simulink model "flattening_3_test"  (Simulink 9.0)
settings: Solver=FixedStepAuto  StartTime=0.0  StopTime=10.0  FixedStep=1.000000  RelTol=1e-3  EnableMultiTasking=on
settings Model: SuppressorTable=22 serialization::archive 11 0 6 0 0 0 0 0  Creator=arnaud  LastModifiedBy=hbourbou
settings DataIOCC: LimitDataPoints=on  SignalLoggingSaveFormat=ModelDataLogs
settings OptimizationCC: ExpressionDepthLimit=2147483647
settings DebuggingCC: SolverPrmCheckMsg=warning  FcnCallInpInsideContextMsg=warning  StateNameClashWarn=warning  StrictBusMsg=Warning
settings GRTTargetCC: CombineOutputUpdateFcns=off  GRTInterface=on

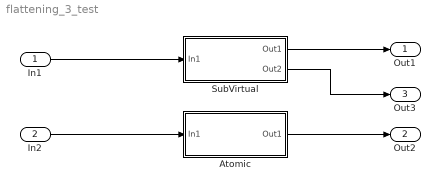
== system flattening_3_test ==
  In1 : Inport
  In2 : Inport  Port=2
  Atomic : Subsystem  TreatAsAtomicUnit=on
  SubVirtual : Subsystem
  Out1 : Outport
  Out2 : Outport  Port=2
  Out3 : Outport  Port=3
  wires:
  SubVirtual/1(Out1) -> Out1/1
  Atomic/1(Out1) -> Out2/1
  In1/1 -> SubVirtual/1(In1)
  In2/1 -> Atomic/1(In1)
  SubVirtual/2(Out2) -> Out3/1

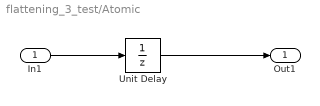
== system flattening_3_test/Atomic ==
  In1 : Inport
  Unit Delay : UnitDelay
  Out1 : Outport
  wires:
  In1/1 -> Unit Delay/1
  Unit Delay/1 -> Out1/1

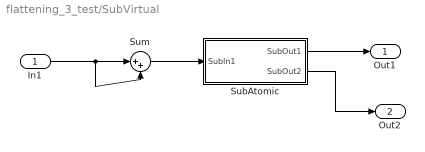
== system flattening_3_test/SubVirtual ==
  In1 : Inport
  SubAtomic : Subsystem  TreatAsAtomicUnit=on
  Sum : Sum  Inputs=|++
  Out1 : Outport
  Out2 : Outport  Port=2
  wires:
  SubAtomic/1(SubOut1) -> Out1/1
  Sum/1 -> SubAtomic/1(SubIn1)
  In1/1 -> Sum/1, Sum/2
  SubAtomic/2(SubOut2) -> Out2/1

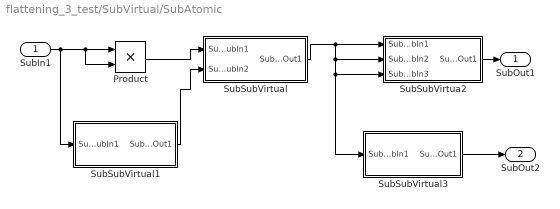
== system flattening_3_test/SubVirtual/SubAtomic ==
  SubIn1 : Inport
  Product : Product  RndMeth=Zero
  SubSubVirtua2 : Subsystem
  SubSubVirtual : Subsystem
  SubSubVirtual1 : Subsystem
  SubSubVirtual3 : Subsystem
  SubOut1 : Outport
  SubOut2 : Outport  Port=2
  wires:
  SubSubVirtual/1(SubSubOut1) -> SubSubVirtua2/1(SubSubIn1), SubSubVirtua2/2(SubSubIn2), SubSubVirtua2/3(SubSubIn3), SubSubVirtual3/1(SubSubIn1)
  Product/1 -> SubSubVirtual/1(SubSubIn1)
  SubIn1/1 -> Product/1, Product/2, SubSubVirtual1/1(SubSubIn1)
  SubSubVirtual1/1(SubSubOut1) -> SubSubVirtual/2(SubSubIn2)
  SubSubVirtua2/1(SubSubOut1) -> SubOut1/1
  SubSubVirtual3/1(SubSubOut1) -> SubOut2/1

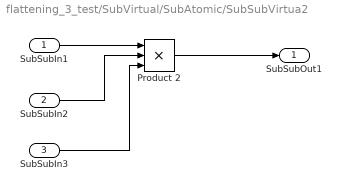
== system flattening_3_test/SubVirtual/SubAtomic/SubSubVirtua2 ==
  SubSubIn1 : Inport
  SubSubIn2 : Inport  Port=2
  SubSubIn3 : Inport  Port=3
  Product 2 : Product  Inputs=3  RndMeth=Zero
  SubSubOut1 : Outport
  wires:
  SubSubIn1/1 -> Product 2/1
  Product 2/1 -> SubSubOut1/1
  SubSubIn2/1 -> Product 2/2
  SubSubIn3/1 -> Product 2/3

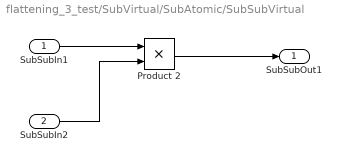
== system flattening_3_test/SubVirtual/SubAtomic/SubSubVirtual ==
  SubSubIn1 : Inport
  SubSubIn2 : Inport  Port=2
  Product 2 : Product  RndMeth=Zero
  SubSubOut1 : Outport
  wires:
  SubSubIn1/1 -> Product 2/1
  Product 2/1 -> SubSubOut1/1
  SubSubIn2/1 -> Product 2/2

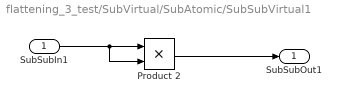
== system flattening_3_test/SubVirtual/SubAtomic/SubSubVirtual1 ==
  SubSubIn1 : Inport
  Product 2 : Product  RndMeth=Zero
  SubSubOut1 : Outport
  wires:
  SubSubIn1/1 -> Product 2/1, Product 2/2
  Product 2/1 -> SubSubOut1/1

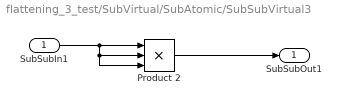
== system flattening_3_test/SubVirtual/SubAtomic/SubSubVirtual3 ==
  SubSubIn1 : Inport
  Product 2 : Product  Inputs=3  RndMeth=Zero
  SubSubOut1 : Outport
  wires:
  SubSubIn1/1 -> Product 2/1, Product 2/2, Product 2/3
  Product 2/1 -> SubSubOut1/1
